simulink model "ABS"  (Simulink 9.2)
settings: Solver=ode45  StartTime=0.0  StopTime=10  RelTol=1e-6
settings Model: Creator=jinwooro  LastModifiedBy=jinwooro
settings DataIOCC: LimitDataPoints=off  SaveFormat=Dataset  SignalLoggingSaveFormat=Dataset
settings OptimizationCC: LifeSpan=auto
settings DebuggingCC: UnderspecifiedInitializationDetection=Simplified  MergeDetectMultiDrivingBlocksExec=error  FcnCallInpInsideContextMsg=error  StateNameClashWarn=none  SFUnexpectedBacktrackingDiag=error  SFNoUnconditionalDefaultTransitionDiag=error  SFExecutionAtInitializationDiag=warning
settings HardwareCC: ProdBitPerPointer=64  ProdBitPerSizeT=64  ProdBitPerPtrDiffT=64  ProdLargestAtomicFloat=Float  ProdIntDivRoundTo=Zero  ProdEndianess=LittleEndian  ProdWordSize=64  ProdHWDeviceType=Intel->x86-64 (Windows64)
settings ModelReferenceCC: PropagateSignalLabelsOutOfModel=on
settings SFSimCC: SimUseLocalCustomCode=on
settings RTWCC: RTWUseLocalCustomCode=on
settings CodeAppCC: StateflowObjectComments=off
settings GRTTargetCC: TargetLangStandard=C99 (ISO)  GeneratePreprocessorConditionals=Use local settings  CombineOutputUpdateFcns=on  GRTInterface=off
settings ConfigComp: CovMetricSettings=dwe  CovHtmlReporting=off  CovSaveCumulativeToWorkspaceVar=off  CovSaveSingleToWorkspaceVar=off  CovExternalEMLEnable=on

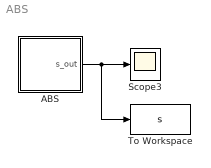
== system ABS ==
  ABS : Stateflow chart  TreatAsAtomicUnit=on
  Scope3 : Scope
  To Workspace : ToWorkspace  VariableName=s  SaveFormat=Timeseries  SampleTime=-1
  wires:
  ABS/1(s_out) -> To Workspace/1, Scope3/1

== stateflow chart ABS ==
  settings: updateMethod=CONTINUOUS
  state Lock
    du:
    s_dot = 0.13;
    s_out = s;
  state Release
    du:
    s_dot = -0.13;
    s_out = s;
  (default) -> Lock : {s = 0;}
  Lock -> Release : [s >= 0.22]
  Release -> Lock : [ s <= 0.18]
  data: s local double; s_out output double
  data s settings: updateMethod=SF_CONTINUOUS_TIME_DATA
